simulink model "LKAS_AutoSave_DF_20220125_0841"  (R2018b)
settings: Solver=FixedStepDiscrete  StartTime=0.0  StopTime=10.0  FixedStep=0.01  RelTol=1e-3
InitFcn:
  | tmpVer = ver('MATLAB');
  | tmpVer = str2num(tmpVer.Version);
  | % -------------------------------------------------------------------
  | %  MATLAB file generated by Simulink.saveVars on 21-Nov-2019 10:06:14
  | %  MATLAB version: 7.13.0.564 (R2011b)
  | % -------------------------------------------------------------------
  | 
  | 
  | SInt16 = Simulink.AliasType;
  | SInt16.Description = 'Num';
  | if (tmpVer > 7.11)
  | 	SInt16.DataScope = 'Auto';
  | end
  | SInt16.HeaderFile = 'Rte_Type.h';
  | SInt16.BaseType = 'int16';
  | 
  | SInt32 = Simulink.AliasType;
  | SInt32.Description = 'Num';
  | if (tmpVer > 7.11)
  | 	SInt32.DataScope = 'Auto';
  | end
  | SInt32.HeaderFile = 'Rte_Type.h';
  | SInt32.BaseType = 'int32';
  | 
  | SInt8 = Simulink.AliasType;
  | SInt8.Description = 'Num';
  | if (tmpVer > 7.11)
  | 	SInt8.DataScope = 'Auto';
  | end
  | SInt8.HeaderFile = 'Rte_Type.h';
  | SInt8.BaseType = 'int8';
  | 
  | T_A_m2_1024_1_u32 = Simulink.NumericType;
  | T_A_m2_1024_1_u32.Description = 'm2 (square meters  (m2))';
  | if (tmpVer > 7.11)
  | 	T_A_m2_1024_1_u32.DataScope = 'Auto';
  | end
  | T_A_m2_1024_1_u32.HeaderFile = 'Rte_Type.h';
  | T_A_m2_1024_1_u32.DataTypeMode = 'Fixed-point: slope and bias scaling';
  | T_A_m2_1024_1_u32.SignednessBool = false;
  | T_A_m2_1024_1_u32.WordLength = 32;
  | T_A_m2_1024_1_u32.FixedExponent = -10;
  | T_A_m2_1024_1_u32.SlopeAdjustmentFactor = 1;
  | T_A_m2_1024_1_u32.Bias = 0;
  | T_A_m2_1024_1_u32.DataTypeOverride = 'Inherit';
  | T_A_m2_1024_1_u32.IsAlias = true;
  | 
  | T_A_m2_65536_1_u16 = Simulink.NumericType;
  | T_A_m2_65536_1_u16.Description = 'm2 (square meters  (m2))';
  | if (tmpVer > 7.11)
  | 	T_A_m2_65536_1_u16.DataScope = 'Auto';
  | end
  | T_A_m2_65536_1_u16.HeaderFile = 'Rte_Type.h';
  | T_A_m2_65536_1_u16.DataTypeMode = 'Fixed-point: slope and bias scaling';
  | T_A_m2_65536_1_u16.SignednessBool = false;
  | T_A_m2_65536_1_u16.WordLength = 16;
  | T_A_m2_65536_1_u16.FixedExponent = -16;
  | T_A_m2_65536_1_u16.SlopeAdjustmentFactor = 1;
  | T_A_m2_65536_1_u16.Bias = 0;
  | T_A_m2_65536_1_u16.DataTypeOverride = 'Inherit';
  | ... (+4647 lines)
StopFcn:
  | clear  T_A_m2_1024_1_u32 T_A_m2_65536_1_u16 T_A_m2_Float32 T_A_mm2_10_1_u16 T_A_mm2_4_1_s16 T_A_mm2_Float32 T_Cnt_Num_10_1_u32 T_Cnt_Num_1_1_s16 T_Cnt_Num_1_1_s32 T_Cnt_Num_1_1_s8 T_Cnt_Num_1_1_u16 T_Cnt_Num_1_1_u32 T_Cnt_Num_1_1_u8 T_E_J_1_1_s32 T_E_J_Float32 T_E_kJ_128_1_s32 T_E_kJ_Float32 T_E_kwh_10_1_u16 T_E_kwh_Float32 T_Epl_kwhpkm_100_1_u16 T_Epl_kwhpkm_Float32 T_F_N_1_1_s16 T_F_N_Float32 T_I_A_1000_1_u16 T_I_A_1048576_1_s32 T_I_A_2048_1_s16 T_I_A_32_1_s16 T_I_A_Float32 T_I_mA_1_1_s16 T_I_mA_32768_128_s16 T_I_mA_Float32 T_J_kgpm2_128_1_u16 T_J_kgpm2_Float32 T_K_NA_1000_1_s16 T_K_NA_100_1_s16 T_K_NA_100_1_u16 T_K_NA_1024_1_s16 T_K_NA_1024_1_u16 T_K_NA_128_1_s16 T_K_NA_128_1_u16 T_K_NA_128_1_u8 T_K_NA_16777216_1_u32 T_K_NA_16_1_s16 T_K_NA_16_1_u16 T_K_NA_16_1_u8 T_K_NA_1_16_u16 T_K_NA_1_1_s16 T_K_NA_1_1_u16 T_K_NA_1_1_u8 T_K_NA_32768_1_s16 T_K_NA_32768_1_u16 T_K_NA_32_1_s8 T_K_NA_4096_1_u16 T_K_NA_4194304_1_s32 T_K_NA_4194304_1_u16 T_K_NA_65536_1_s32 T_K_NA_65536_1_u16 T_K_NA_8192_1_s16 T_K_NA_8_1_s16 T_K_NA_Float32 T_M_Nm_16_1_s16 T_M_Nm_1_1_s16 T_M_Nm_32768_1_s16 T_M_Nm_32_1_s16 T_M_Nm_4_1_s16 T_M_Nm_512_1_s16 T_M_Nm_Float32 T_P_W_1_4_s16 T_P_W_1_8_s16 T_P_W_Float32 T_P_kW_128_1_s16 T_P_kW_1_8_s16 T_P_kW_8_1_s32 T_P_kW_Float32 T_Pct_pct_1024_1_s32 T_Pct_pct_1024_1_u32 T_Pct_pct_10_1_s16 T_Pct_pct_10_1_u32 T_Pct_pct_128_100_s8 T_Pct_pct_1_1_s16 T_Pct_pct_1_4_u8 T_Pct_pct_255_100_u16 T_Pct_pct_255_100_u8 T_Pct_pct_256_1_s16 T_Pct_pct_256_1_u16 T_Pct_pct_65535_100_u16 T_Pct_pct_Float32 T_R_ohm_1024_1_s16 T_R_ohm_32_1_s16 T_R_ohm_Float32 T_TK_K_16_1_s16 T_TK_K_Float32 T_T_degC_10_400_1_u16 T_T_degC_16_1_s16 T_T_degC_1_40_1_u8 T_T_degC_2_80_1_u8 T_T_degC_Float32 T_U_V_1000_1_u16 T_U_V_10_1_u8 T_U_V_200_1_u8 T_U_V_32_1_s16 T_U_V_4096_1_s16 T_U_V_512_1_s16 T_U_V_65535_8_u16 T_U_V_8192_1_u16 T_U_V_Float32 T_U_mV_1_1_s16 T_U_mV_256_20_u16 T_U_mV_Float32 T_V_l_256_1_s16 T_V_l_4096_1_s16 T_V_l_64_1_s16 T_V_l_65535_100_u16 T_V_l_Float32 T_V_ml_128_1_s16 T_V_ml_1_1_s16 T_V_ml_32768_1_s16 T_V_ml_Float32 T_V_ul_32_1_u16 T_V_ul_Float32 T_Vpl_clpkm_512_1_u16 T_Vpl_clpkm_Float32 T_a_kphps_16_1_s16 T_a_kphps_Float32 T_a_mps2_128_1_s16 T_a_mps2_Float32 T_c_MJpkg_256_1_s16 T_c_MJpkg_Float32 T_c_kJpgpK_1024_1_s16 T_c_kJpgpK_Float32 T_c_kJpkgpK_128_1_u16 T_c_kJpkgpK_Float32 T_chrg_Ah_1_1_s16 T_chrg_Ah_1_1_u16 T_chrg_Ah_1_1_u8 T_chrg_Ah_256_1_u16 T_chrg_Ah_4194304_1_s32 T_chrg_Ah_512_1_u16 T_chrg_Ah_8_1_u16 T_chrg_Ah_Float32 T_cmp_NA_100_1_s16 T_cmp_NA_128_1_s16 T_cmp_NA_16_1_s16 T_cmp_NA_32768_1_u16 T_cmp_NA_Float32 T_d2n_rpmps2_4_1_s16 T_d2n_rpmps2_Float32 T_dPct_pctps_16_1_s16 T_dPct_pctps_256_1_s16 T_dPct_pctps_Float32 T_dT_degCps_128_1_s16 T_dT_degCps_Float32 T_dV_lph_1_1_s16 T_dV_lph_Float32 T_dV_lpm_128_1_s16 T_dV_lpm_32_1_s16 T_dV_lpm_Float32 T_dV_lps_1024_1_u16 T_dV_lps_4_1_u16 T_dV_lps_Float32 T_dV_mlps_1024_1_s16 T_dV_mlps_Float32 T_d_BitField16 T_dm_gps_128_1_s16 T_dm_gps_128_1_u16 T_dm_gps_256_1_u16 T_dm_gps_Float32 T_dm_mgps_1_1_s16 T_dm_mgps_Float32 T_dn_rpmps_1_1_s16 T_dn_rpmps_2_1_s16 T_dn_rpmps_Float32 T_dp_Paps_1_1_s16 T_dp_Paps_Float32 T_dp_kPaps_1_1_s16 T_dp_kPaps_8_1_s16 T_dp_kPaps_Float32 T_dphi_degps_128_1_s16 T_dphi_degps_8_1_s16 T_dphi_degps_Float32 T_dr_ps_256_1_s16 T_dr_ps_Float32 T_drho_mgplps_1_2_s16 T_drho_mgplps_Float32 T_e_NA_1_1_u8 T_f_Hz_1_1_u16 T_f_Hz_1_1_u32 T_f_Hz_64_1_u16 T_f_Hz_8_1_s16 T_f_Hz_Float32 T_g_BitField32 T_l_km_16_1_s16 T_l_km_1_1_u16 T_l_km_1_1_u32 T_l_km_Float32 T_l_m_1024_1_s16 T_l_m_16_1_s16 T_l_m_1_1_u32 T_l_m_Float32 T_l_mm_16_1_s16 T_l_mm_1_1_u16 T_l_mm_4096_1_s16 T_l_mm_4_1_u8 T_l_mm_64_1_s16 T_l_mm_Float32 T_m_g_1_1_s16 T_m_g_2048_1_s16 T_m_g_32_1_u16 T_m_g_Float32 T_m_kg_1024_1_s16 T_m_kg_1_1_s16 T_m_kg_1_1_u32 T_m_kg_Float32 T_m_mg_128_1_s16 T_m_mg_32_1_s16 T_m_mg_Float32 T_n_rpm_1_1_s16 T_n_rpm_1_25_u8 T_n_rpm_256_50_u16 T_n_rpm_2_25_u8 T_n_rpm_4_1_u16 T_n_rpm_Float32 T_p_MPa_64_1_s16 T_p_MPa_Float32 T_p_Pa_1_1_s16 T_p_Pa_Float32 T_p_kPa_1_10_u16 T_p_kPa_1_1_s16 T_p_kPa_1_1_u8 T_p_kPa_256_1_u16 T_p_kPa_32_1_u16 T_p_kPa_64_1_s16 T_p_kPa_Float32 T_phi_deg_100_1_s16 T_phi_deg_1024_1_s16 T_phi_deg_128_1_s16 T_phi_deg_1_1_u8 T_phi_deg_256_1_s16 T_phi_deg_2_1_s8 T_phi_deg_32_1_s16 T_phi_deg_512_6_s32 T_phi_deg_Float32 T_phi_rad_2048_1_s16 T_phi_rad_Float32 T_r_NA_1024_1_s16 T_r_NA_1024_1_u16 T_r_NA_16384_1_s16 T_r_NA_16_1_s16 T_r_NA_256_1_s8 T_r_NA_256_1_u16 T_r_NA_32768_1_u16 T_r_NA_32_1_u16 T_r_NA_4096_1_s16 T_r_NA_65535_2_u16 T_r_NA_8192_1_u16 T_r_NA_Float32 T_rho_gpl_8192_1_s16 T_rho_gpl_Float32 T_rho_kgpm3_16_1_s16 T_rho_kgpm3_Float32 T_rho_mgpl_1_1_s16 T_rho_mgpl_64_1_s16 T_rho_mgpl_Float32 T_t_hour_1_1_s16 T_t_hour_Float32 T_t_m_1_1_u16 T_t_m_Float32 T_t_ms_1_1_s16 T_t_ms_1_1_u16 T_t_ms_1_1_u32 T_t_ms_4096_1_s16 T_t_ms_64_1_s16 T_t_ms_Float32 T_t_s_1000_1_s16 T_t_s_100_1_s16 T_t_s_10_1_s16 T_t_s_10_1_u16 T_t_s_1_1_s16 T_t_s_1_1_u16 T_t_s_1_1_u32 T_t_s_Float32 T_t_us_10_1_u32 T_t_us_1_1_s16 T_t_us_1_1_u32 T_t_us_1_4_u16 T_t_us_Float32 T_v_kph_1_1_u8 T_v_kph_64_1_s16 T_v_kph_64_1_u16 T_v_kph_Float32 T_v_mps_256_1_s16 T_v_mps_Float32 T_w_radps_32_1_s16 T_w_radps_Float32 T_y_BitField8 T_y_BitFieldDiagProgress T_y_BitFieldDiagStatus T_y_NA_1_1_u8 SInt16 SInt32 SInt8 T_BOOLEAN UInt16 UInt32 UInt8 s16 s32 s8 u16 u32 u8
model workspace (MAT data in the model file):
  MCOS : class17 (value not decoded)
  MCOS : class17 (value not decoded)
  MCOS : class17 (value not decoded)
  MCOS : class17 (value not decoded)
  MCOS : class17 (value not decoded)
  MCOS : class17 (value not decoded)
  MCOS : class17 (value not decoded)
  MCOS : class17 (value not decoded)
  MCOS : class17 (value not decoded)
  MCOS : class17 (value not decoded)
  MCOS : class17 (value not decoded)
  MCOS : class17 (value not decoded)
  MCOS : class17 (value not decoded)
  MCOS : class17 (value not decoded)
  MCOS : class17 (value not decoded)
  MCOS : class17 (value not decoded)
  MCOS : class17 (value not decoded)
  MCOS : class17 (value not decoded)
  MCOS : class17 (value not decoded)
  MCOS : class17 (value not decoded)
  MCOS : class17 (value not decoded)
  MCOS : class17 (value not decoded)
  MCOS : class17 (value not decoded)
  MCOS : class17 (value not decoded)
  MCOS : class17 (value not decoded)
  MCOS : class17 (value not decoded)
  MCOS : class17 (value not decoded)
  MCOS : class17 (value not decoded)
  MCOS : class17 (value not decoded)
  MCOS : class17 (value not decoded)
  MCOS : class17 (value not decoded)
  MCOS : class17 (value not decoded)
  MCOS : class17 (value not decoded)
  MCOS : class17 (value not decoded)
  MCOS : class17 (value not decoded)
  MCOS : class17 (value not decoded)
  MCOS : class17 (value not decoded)
  MCOS : class17 (value not decoded)
  MCOS : class17 (value not decoded)
  MCOS : class17 (value not decoded)
  MCOS : class17 (value not decoded)
  MCOS : class17 (value not decoded)
  MCOS : class17 (value not decoded)
  MCOS : class17 (value not decoded)
  MCOS : class17 (value not decoded)
  MCOS : class17 (value not decoded)
  MCOS : class17 (value not decoded)
  MCOS : class17 (value not decoded)
  MCOS : class17 (value not decoded)
  MCOS : class17 (value not decoded)
  MCOS : class17 (value not decoded)
  MCOS : class17 (value not decoded)
  MCOS : class17 (value not decoded)
  MCOS : class17 (value not decoded)
  MCOS : class17 (value not decoded)
  MCOS : class17 (value not decoded)
  MCOS : class17 (value not decoded)
  MCOS : class17 (value not decoded)
  MCOS : class17 (value not decoded)
  MCOS : class17 (value not decoded)
  MCOS : class17 (value not decoded)
  MCOS : class17 (value not decoded)
  MCOS : class17 (value not decoded)
  MCOS : class17 (value not decoded)
  MCOS : class17 (value not decoded)
  MCOS : class17 (value not decoded)
  MCOS : class17 (value not decoded)
  MCOS : class17 (value not decoded)
  MCOS : class17 (value not decoded)
  MCOS : class17 (value not decoded)
  MCOS : class17 (value not decoded)
  MCOS : class17 (value not decoded)
  MCOS : class17 (value not decoded)
  MCOS : class17 (value not decoded)
  MCOS : class17 (value not decoded)
  MCOS : class17 (value not decoded)
  MCOS : class17 (value not decoded)
  MCOS : class17 (value not decoded)
  MCOS : class17 (value not decoded)
  MCOS : class17 (value not decoded)
  MCOS : class17 (value not decoded)
  MCOS : class17 (value not decoded)
  MCOS : class17 (value not decoded)
  MCOS : class17 (value not decoded)
  MCOS : class17 (value not decoded)
  MCOS : class17 (value not decoded)
  MCOS : class17 (value not decoded)
  MCOS : class17 (value not decoded)
  MCOS : class17 (value not decoded)
  MCOS : class17 (value not decoded)
  MCOS : class17 (value not decoded)
  MCOS : class17 (value not decoded)
  MCOS : class17 (value not decoded)
  MCOS : class17 (value not decoded)
  MCOS : class17 (value not decoded)
  MCOS : class17 (value not decoded)
  MCOS : class17 (value not decoded)
  MCOS : class17 (value not decoded)
  MCOS : class17 (value not decoded)
  MCOS : class17 (value not decoded)
  MCOS : class17 (value not decoded)
  MCOS : class17 (value not decoded)
undefined symbols (not defined in the file): LKA_CarWidth, LKA_SampleTime, LKA_StrRatio_C, LKA_Veh2CamL_C, LKA_Veh2CamW_C, LKA_WhlBaseL_C, LL_CompHdAg_C, LL_CompSWA_C, LL_CrvtPrvwT_C, LL_DesDvt_C, LL_DvtComp_C, LL_DvtPrvwT_C, LL_DvtSpdDet_vDvtSpdMin_C, LL_HandsOff_ExitTime, LL_HandsOff_TextTime, LL_HandsOff_WarnTime, LL_HdAgExT_C, LL_HdAgPrvwT_C, LL_LAccMax_C, LL_LAccRMax_C, LL_LDW_EarliestWarnLine_C, LL_LDW_LatestWarnLine_C, LL_LDWS_SUPPRESS_HEADING, LL_LFClb_TFC_FfCtlRatio_C, LL_LFClb_TFC_KdBalance_C, LL_LFClb_TFC_KdMaxSWA_C, LL_LFClb_TFC_KdV1_C, LL_LFClb_TFC_KdV2_C, LL_LFClb_TFC_KdVehSpdLwr_C, LL_LFClb_TFC_KdVehSpdUpr_C, LL_LFClb_TFC_Ki_C, LL_LFClb_TFC_KiMaxSWA_C, LL_LFClb_TFC_Kp_C, LL_LFClb_TFC_KpKlat_C, LL_LFClb_TFC_KpV1_C, LL_LFClb_TFC_KpV2_C, LL_LFClb_TFC_KpVehSpdLwr_C, LL_LFClb_TFC_KpVehSpdUpr_C, LL_LFClb_TFC_PrvwT_C, LL_LKA_EarliestWarnLine_C, LL_LKA_LatestWarnLine_C, LL_LKAExPrcs_ExitC0Dvt, LL_LKAExPrcs_ExitC0Swt, LL_LKAExPrcs_tiExitTime1, LL_LKAExPrcs_tiExitTime2, LL_LKAExPrcs_tiExitTime3, LL_LKAS_OUT_OF_CONTROL_LAT_VEL, LL_LKAS_OUT_OF_CONTROL_TTLC, LL_LKASWASyn_M0, LL_LKASWASyn_M1, LL_LKASWASyn_M2, LL_LKASWASyn_M3K, LL_LKASWASyn_SWAaddMax, LL_LKASWASyn_T2, LL_LKASWASyn_tiTrqSwaRtTime, LL_LKASWASyn_tiTrqSwaTime, LL_LKASWASyn_TrqMax, LL_LKASWASyn_TrqSwaAddSwt, LL_LKASWASyn_TrqSwaRateDiff, LL_LSpdCompT_C ... (+43)
libraries: simulink x136, canmsglib x8, dspstat3 x3, simulink_extras x1
(part 12 of 20)

== system LKAS_AutoSave_DF_20220125_0841/LKAS/LL/LLOn/LKA/LKA Motion Planning (LKAMP) /LKA Motion Planning Calculation (LKAMPCal)/Time Division (TDiv)3 ==
  TDiv_bsTDivInfoOut1 : Inport
  Add : Sum  OutDataTypeStr=uint16
  Constant : Constant  OutDataTypeStr=uint16  SampleTime=-1
  Constant19 : Constant  OutDataTypeStr=uint16  SampleTime=-1
  If : If  NumInputs=2  IfExpression=u1==u2
  Memory : Memory  InheritSampleTime=on
  Merge1 : Merge
  Saturation1 : Saturate  UpperLimit=100  LowerLimit=0  OutDataTypeStr=uint16
      settings: AttributesFormatString="Min = %<LowerLimit>  Max = %<UpperLimit>"
  if action 3 : Subsystem  TreatAsAtomicUnit=on
  if action 4 : Subsystem  TreatAsAtomicUnit=on
  Out2 : Outport
  wires:
  Merge1/1 -> Out2/1
  TDiv_bsTDivInfoOut1/1 -> if action 3/1(In1)
  if action 4/1(Out1) -> Merge1/1
  if action 3/1(Out1) -> Merge1/2
  If/2 -> if action 3/Action
  Saturation1/1 -> If/1
  Add/1 -> Saturation1/1, Memory/1
  Constant19/1 -> If/2
  Constant/1 -> Add/1
  Memory/1 -> Add/2
  If/1 -> if action 4/Action

== system LKAS_AutoSave_DF_20220125_0841/LKAS/LL/LLOn/LKA/LKA Motion Planning (LKAMP) /LKA Motion Planning Calculation (LKAMPCal)/Time Division (TDiv)4 ==
  TDiv_bsTDivInfoOut1 : Inport
  Add : Sum  OutDataTypeStr=uint16
  Constant : Constant  OutDataTypeStr=uint16  SampleTime=-1
  Constant19 : Constant  OutDataTypeStr=uint16  SampleTime=-1
  If : If  NumInputs=2  IfExpression=u1==u2
  Memory : Memory  InheritSampleTime=on
  Merge1 : Merge
  Saturation1 : Saturate  UpperLimit=100  LowerLimit=0  OutDataTypeStr=uint16
      settings: AttributesFormatString="Min = %<LowerLimit>  Max = %<UpperLimit>"
  if action 3 : Subsystem  TreatAsAtomicUnit=on
  if action 4 : Subsystem  TreatAsAtomicUnit=on
  Out2 : Outport
  wires:
  If/1 -> if action 4/Action
  Memory/1 -> Add/2
  Constant/1 -> Add/1
  Constant19/1 -> If/2
  Add/1 -> Memory/1, Saturation1/1
  Saturation1/1 -> If/1
  If/2 -> if action 3/Action
  if action 3/1(Out1) -> Merge1/2
  if action 4/1(Out1) -> Merge1/1
  TDiv_bsTDivInfoOut1/1 -> if action 3/1(In1)
  Merge1/1 -> Out2/1

== system LKAS_AutoSave_DF_20220125_0841/LKAS/LL/LLOn/LKA/LKA Motion Planning (LKAMP) /Motion Planning Input Processing (MPInP)/Lane Information Selection (LaneInfoSel) ==
  LaneInfoSel_stLKAActvFlg : Inport
  LaneInfoSel_facmLftLane : Inport  Port=2
  LaneInfoSel_facmRgtLane : Inport  Port=3
  If : If  IfExpression=u1==1  ElseIfExpressions=u1==2
  If Action Subsystem1 : Subsystem  TreatAsAtomicUnit=on
  If Action Subsystem2 : Subsystem  TreatAsAtomicUnit=on
  If Action Subsystem3 : Subsystem  TreatAsAtomicUnit=on
  Merge : Merge  Inputs=3
  LaneInfoSel_facmActvLane : Outport
  wires:
  LaneInfoSel_facmRgtLane/1 -> If Action Subsystem1/1(In1)
  LaneInfoSel_facmLftLane/1 -> If Action Subsystem2/1(In1)
  LaneInfoSel_stLKAActvFlg/1 -> If/1
  If/1 -> If Action Subsystem2/Action
  If Action Subsystem2/1(Out1) -> Merge/1
  Merge/1 -> LaneInfoSel_facmActvLane/1
  If/2 -> If Action Subsystem1/Action
  If Action Subsystem1/1(Out1) -> Merge/2
  If Action Subsystem3/1(Out1) -> Merge/3
  If/3 -> If Action Subsystem3/Action

== system LKAS_AutoSave_DF_20220125_0841/LKAS/LL/LLOn/LKA/LKA Motion Planning (LKAMP) /Motion Planning Input Processing (MPInP)/Lane Information Selection (LaneInfoSel)1 ==
  LaneInfoSel_stLKAActvFlg : Inport
  LaneInfoSel_facmLftLane : Inport  Port=2
  LaneInfoSel_facmRgtLane : Inport  Port=3
  If : If  IfExpression=u1==1  ElseIfExpressions=u1==2
  If Action Subsystem1 : Subsystem  TreatAsAtomicUnit=on
  If Action Subsystem2 : Subsystem  TreatAsAtomicUnit=on
  If Action Subsystem3 : Subsystem  TreatAsAtomicUnit=on
  Merge : Merge  Inputs=3
  LaneInfoSel_facmActvLane : Outport
  wires:
  LaneInfoSel_facmRgtLane/1 -> If Action Subsystem1/1(In1)
  LaneInfoSel_facmLftLane/1 -> If Action Subsystem2/1(In1)
  LaneInfoSel_stLKAActvFlg/1 -> If/1
  If/1 -> If Action Subsystem2/Action
  If Action Subsystem2/1(Out1) -> Merge/1
  Merge/1 -> LaneInfoSel_facmActvLane/1
  If/2 -> If Action Subsystem1/Action
  If Action Subsystem1/1(Out1) -> Merge/2
  If Action Subsystem3/1(Out1) -> Merge/3
  If/3 -> If Action Subsystem3/Action

== system LKAS_AutoSave_DF_20220125_0841/LKAS/LL/LLOn/LKA/LKA Motion Planning (LKAMP) /Motion Planning Input Processing (MPInP)/Lane Information Selection (LaneInfoSel)2 ==
  LaneInfoSel_stLKAActvFlg : Inport
  LaneInfoSel_facmLftLane : Inport  Port=2
  LaneInfoSel_facmRgtLane : Inport  Port=3
  If : If  IfExpression=u1==1  ElseIfExpressions=u1==2
  If Action Subsystem1 : Subsystem  TreatAsAtomicUnit=on
  If Action Subsystem2 : Subsystem  TreatAsAtomicUnit=on
  If Action Subsystem3 : Subsystem  TreatAsAtomicUnit=on
  Merge : Merge  Inputs=3
  LaneInfoSel_facmActvLane : Outport
  wires:
  LaneInfoSel_facmRgtLane/1 -> If Action Subsystem1/1(In1)
  LaneInfoSel_facmLftLane/1 -> If Action Subsystem2/1(In1)
  LaneInfoSel_stLKAActvFlg/1 -> If/1
  If/1 -> If Action Subsystem2/Action
  If Action Subsystem2/1(Out1) -> Merge/1
  Merge/1 -> LaneInfoSel_facmActvLane/1
  If/2 -> If Action Subsystem1/Action
  If Action Subsystem1/1(Out1) -> Merge/2
  If Action Subsystem3/1(Out1) -> Merge/3
  If/3 -> If Action Subsystem3/Action

== system LKAS_AutoSave_DF_20220125_0841/LKAS/LL/LLOn/LKA/LKA Motion Planning (LKAMP) /Motion Planning Input Processing (MPInP)/Signal Latching ==
  In : Inport
  Add : Sum  OutDataTypeStr=uint16
  Constant : Constant  OutDataTypeStr=uint16  SampleTime=-1
  Constant2 : Constant  Value=LatchTime  OutDataTypeStr=uint16  SampleTime=-1
  If : If  NumInputs=2  IfExpression=u1==u2  ShowElse=off
  Memory : Memory  InheritSampleTime=on
  Saturation1 : Saturate  UpperLimit=10000  LowerLimit=0  OutDataTypeStr=uint16
  "if action " : Subsystem  TreatAsAtomicUnit=on
  Out : Outport
  wires:
  Constant2/1 -> If/2
  In/1 -> "if action "/1(In)
  "if action "/1(Out) -> Out/1
  If/1 -> "if action "/Action
  Constant/1 -> Add/1
  Add/1 -> Memory/1, Saturation1/1
  Memory/1 -> Add/2
  Saturation1/1 -> If/1

== system LKAS_AutoSave_DF_20220125_0841/LKAS/LL/LLOn/LKA/LKA Motion Planning (LKAMP) /Motion Planning Input Processing (MPInP)/Signal Latching2 ==
  In : Inport
  Add : Sum  OutDataTypeStr=uint16
  Constant : Constant  OutDataTypeStr=uint16  SampleTime=-1
  Constant2 : Constant  Value=LatchTime  OutDataTypeStr=uint16  SampleTime=-1
  If : If  NumInputs=2  IfExpression=u1==u2  ShowElse=off
  Memory : Memory  InheritSampleTime=on
  Saturation1 : Saturate  UpperLimit=10000  LowerLimit=0  OutDataTypeStr=uint16
  "if action " : Subsystem  TreatAsAtomicUnit=on
  Out : Outport
  wires:
  Constant2/1 -> If/2
  In/1 -> "if action "/1(In)
  "if action "/1(Out) -> Out/1
  If/1 -> "if action "/Action
  Constant/1 -> Add/1
  Add/1 -> Saturation1/1
  Memory/1 -> Add/2
  Saturation1/1 -> Memory/1, If/1

== system LKAS_AutoSave_DF_20220125_0841/LKAS/LL/LLOn/LKA/LKA Motion Planning (LKAMP) /Motion Planning Input Processing (MPInP)/Signal Latching3 ==
  In : Inport
  Add : Sum  OutDataTypeStr=uint16
  Constant : Constant  OutDataTypeStr=uint16  SampleTime=-1
  Constant2 : Constant  Value=LatchTime  OutDataTypeStr=uint16  SampleTime=-1
  If : If  NumInputs=2  IfExpression=u1==u2  ShowElse=off
  Memory : Memory  InheritSampleTime=on
  Saturation1 : Saturate  UpperLimit=10000  LowerLimit=0  OutDataTypeStr=uint16
  "if action " : Subsystem  TreatAsAtomicUnit=on
  Out : Outport
  wires:
  Saturation1/1 -> If/1, Memory/1
  Memory/1 -> Add/2
  Add/1 -> Saturation1/1
  Constant/1 -> Add/1
  If/1 -> "if action "/Action
  "if action "/1(Out) -> Out/1
  In/1 -> "if action "/1(In)
  Constant2/1 -> If/2

== system LKAS_AutoSave_DF_20220125_0841/LKAS/LL/LLOn/LKA/LKA Motion Planning (LKAMP) /Motion Planning Input Processing (MPInP)/Signal Latching4 ==
  In : Inport
  Add : Sum  OutDataTypeStr=uint16
  Constant : Constant  OutDataTypeStr=uint16  SampleTime=-1
  Constant2 : Constant  Value=LatchTime  OutDataTypeStr=uint16  SampleTime=-1
  If : If  NumInputs=2  IfExpression=u1==u2  ShowElse=off
  Memory : Memory  InheritSampleTime=on
  Saturation1 : Saturate  UpperLimit=10000  LowerLimit=0  OutDataTypeStr=uint16
  "if action " : Subsystem  TreatAsAtomicUnit=on
  Out : Outport
  wires:
  Constant2/1 -> If/2
  In/1 -> "if action "/1(In)
  "if action "/1(Out) -> Out/1
  If/1 -> "if action "/Action
  Constant/1 -> Add/1
  Add/1 -> Saturation1/1
  Memory/1 -> Add/2
  Saturation1/1 -> Memory/1, If/1

== system LKAS_AutoSave_DF_20220125_0841/LKAS/LL/LLOn/LKA/LKA Motion Planning (LKAMP) /Motion Planning Input Processing (MPInP)/Signal Latching5 ==
  In : Inport
  Add : Sum  OutDataTypeStr=uint16
  Constant : Constant  OutDataTypeStr=uint16  SampleTime=-1
  Constant2 : Constant  Value=LatchTime  OutDataTypeStr=uint16  SampleTime=-1
  If : If  NumInputs=2  IfExpression=u1==u2  ShowElse=off
  Memory : Memory  InheritSampleTime=on
  Saturation1 : Saturate  UpperLimit=10000  LowerLimit=0  OutDataTypeStr=uint16
  "if action " : Subsystem  TreatAsAtomicUnit=on
  Out : Outport
  wires:
  Constant2/1 -> If/2
  In/1 -> "if action "/1(In)
  "if action "/1(Out) -> Out/1
  If/1 -> "if action "/Action
  Constant/1 -> Add/1
  Add/1 -> Saturation1/1
  Memory/1 -> Add/2
  Saturation1/1 -> Memory/1, If/1

== system LKAS_AutoSave_DF_20220125_0841/LKAS/LL/LLOn/LKA/LKA Motion Planning (LKAMP) /Motion Planning Input Processing (MPInP)/Signal Latching6 ==
  In : Inport
  Add : Sum  OutDataTypeStr=uint16
  Constant : Constant  OutDataTypeStr=uint16  SampleTime=-1
  Constant2 : Constant  Value=LatchTime  OutDataTypeStr=uint16  SampleTime=-1
  If : If  NumInputs=2  IfExpression=u1==u2  ShowElse=off
  Memory : Memory  InheritSampleTime=on
  Saturation1 : Saturate  UpperLimit=10000  LowerLimit=0  OutDataTypeStr=uint16
  "if action " : Subsystem  TreatAsAtomicUnit=on
  Out : Outport
  wires:
  Constant2/1 -> If/2
  In/1 -> "if action "/1(In)
  "if action "/1(Out) -> Out/1
  If/1 -> "if action "/Action
  Constant/1 -> Add/1
  Add/1 -> Saturation1/1
  Memory/1 -> Add/2
  Saturation1/1 -> Memory/1, If/1

== system LKAS_AutoSave_DF_20220125_0841/LKAS/LL/LLOn/LKA/LKA Motion Planning (LKAMP) /Motion Planning Input Processing (MPInP)/Signal Latching7 ==
  In : Inport
  Add : Sum  OutDataTypeStr=uint16
  Constant : Constant  OutDataTypeStr=uint16  SampleTime=-1
  Constant2 : Constant  Value=LatchTime  OutDataTypeStr=uint16  SampleTime=-1
  If : If  NumInputs=2  IfExpression=u1==u2  ShowElse=off
  Memory : Memory  InheritSampleTime=on
  Saturation1 : Saturate  UpperLimit=10000  LowerLimit=0  OutDataTypeStr=uint16
  "if action " : Subsystem  TreatAsAtomicUnit=on
  Out : Outport
  wires:
  Saturation1/1 -> If/1, Memory/1
  Memory/1 -> Add/2
  Add/1 -> Saturation1/1
  Constant/1 -> Add/1
  If/1 -> "if action "/Action
  "if action "/1(Out) -> Out/1
  In/1 -> "if action "/1(In)
  Constant2/1 -> If/2

== system LKAS_AutoSave_DF_20220125_0841/LKAS/LL/LLOn/LKA/LKA Motion Planning (LKAMP) /Motion Planning Input Processing (MPInP)/Subsystem ==
  In1 : Inport
  If : If  IfExpression=u1==1  ElseIfExpressions=u1==2
  If Action Subsystem1 : Subsystem  TreatAsAtomicUnit=on
  If Action Subsystem2 : Subsystem  TreatAsAtomicUnit=on
  If Action Subsystem3 : Subsystem  TreatAsAtomicUnit=on
  Merge : Merge  Inputs=3
  Out6 : Outport
  wires:
  If/3 -> If Action Subsystem3/Action
  If Action Subsystem3/1(Out1) -> Merge/3
  If Action Subsystem1/1(Out1) -> Merge/2
  If/2 -> If Action Subsystem1/Action
  Merge/1 -> Out6/1
  If Action Subsystem2/1(Out1) -> Merge/1
  If/1 -> If Action Subsystem2/Action
  In1/1 -> If/1

== system LKAS_AutoSave_DF_20220125_0841/LKAS/LL/LLOn/LKA/LKA Motion Planning (LKAMP) /Switching Condition (SwtCon)/Ending Heading Angle Determination (EndHdAgDet) ==
  EndHdAgDet_stLKAActvFlg : Inport
  EndHdAgDet_vVehSpd : Inport  Port=2
  EndHdAgDet_crPrvwCrvt : Inport  Port=3
  EndHdAgDet_lLaneWidth_C : Inport  Port=4
  EndHdAgDet_lCarWidth_C : Inport  Port=5
  EndHdAgDet_tiHdAgExTime_C : Inport  Port=6
  EndHdAgDet_tiLSpdCompT_C : Inport  Port=7
  Add : Sum  Inputs=+-  OutDataTypeStr=single
  Add1 : Sum  OutDataTypeStr=single
  Divide : Product  Inputs=/*  OutDataTypeStr=single
  Divide1 : Product  Inputs=*/  OutDataTypeStr=single
  Lateral Speed Compensation (LSpdComp) : Subsystem
  kph To mps : Gain  Gain=1/3.6  OutDataTypeStr=single
  EndHdAgDet_phiHdAgMax : Outport
  wires:
  EndHdAgDet_tiLSpdCompT_C/1 -> Lateral Speed Compensation (LSpdComp)/4(LSpdComp_tiLSpdCompT_C)
  EndHdAgDet_crPrvwCrvt/1 -> Lateral Speed Compensation (LSpdComp)/3(LSpdComp_crPrvwCrvt)
  Add1/1 -> EndHdAgDet_phiHdAgMax/1
  Divide1/1 -> Add1/1
  Lateral Speed Compensation (LSpdComp)/1(LSpdComp_phiLSpdComp) -> Add1/2
  Add/1 -> Divide/2
  EndHdAgDet_stLKAActvFlg/1 -> Lateral Speed Compensation (LSpdComp)/2(LSpdComp_stLKAFlg)
  EndHdAgDet_vVehSpd/1 -> kph To mps/1
  EndHdAgDet_tiHdAgExTime_C/1 -> Divide/1
  kph To mps/1 -> Divide1/2, Lateral Speed Compensation (LSpdComp)/1(LSpdComp_vVehSpd)
  EndHdAgDet_lCarWidth_C/1 -> Add/2
  EndHdAgDet_lLaneWidth_C/1 -> Add/1
  Divide/1 -> Divide1/1

== system LKAS_AutoSave_DF_20220125_0841/LKAS/LL/LLOn/LKA/LKA Motion Planning (LKAMP) /Switching Condition (SwtCon)/If Action Subsystem ==
  In1 : Inport
  Action Port : ActionPort  InitializeStates=reset
      settings: AttributesFormatString=states = %<InitializeStates>
  Gain2 : Gain  Gain=-1  OutDataTypeStr=Inherit: Same as input
  Out1 : Outport
      settings: AttributesFormatString=%<OutputWhenDisabled> = %<InitialOutput>
  wires:
  In1/1 -> Gain2/1
  Gain2/1 -> Out1/1  "HdAgMax"

== system LKAS_AutoSave_DF_20220125_0841/LKAS/LL/LLOn/LKA/LKA Motion Planning (LKAMP) /Switching Condition (SwtCon)/If Action Subsystem1 ==
  In1 : Inport
  Action Port : ActionPort  InitializeStates=reset
      settings: AttributesFormatString=states = %<InitializeStates>
  Cast To Single1 : DataTypeConversion  LockScale=on
  Out1 : Outport
      settings: AttributesFormatString=%<OutputWhenDisabled> = %<InitialOutput>
  wires:
  In1/1 -> Cast To Single1/1
  Cast To Single1/1 -> Out1/1  "HdAgMax"

== system LKAS_AutoSave_DF_20220125_0841/LKAS/LL/LLOn/LKA/LKA Motion Planning (LKAMP) /Switching Condition (SwtCon)/If Action Subsystem2 ==
  Action Port : ActionPort  InitializeStates=reset
      settings: AttributesFormatString=states = %<InitializeStates>
  Constant2 : Constant  Value=0  OutDataTypeStr=single  SampleTime=-1
  Out1 : Outport
      settings: AttributesFormatString=%<OutputWhenDisabled> = %<InitialOutput>
  wires:
  Constant2/1 -> Out1/1  "HdAgMax"

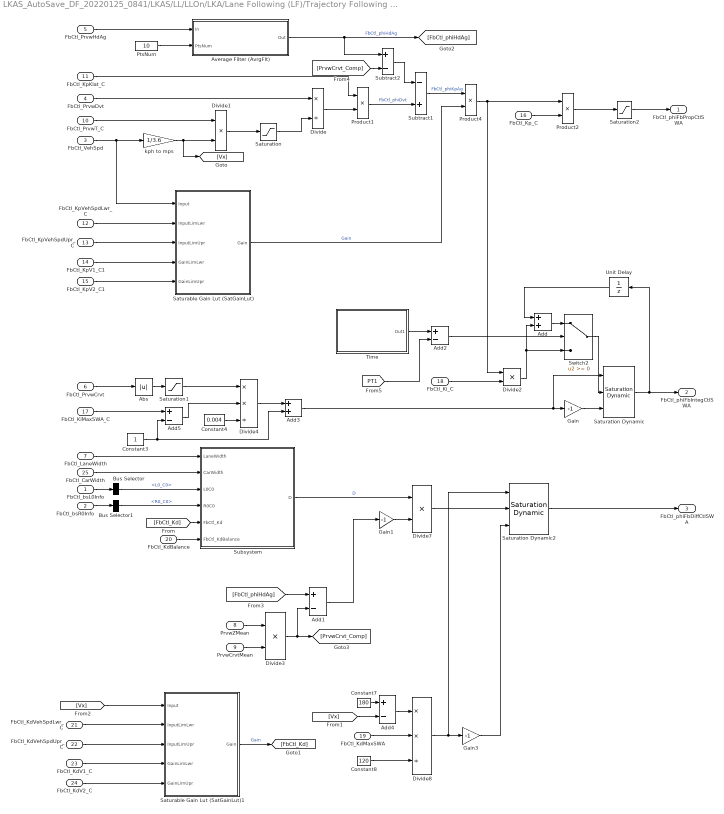
== system LKAS_AutoSave_DF_20220125_0841/LKAS/LL/LLOn/LKA/Lane Following (LF)/Trajectory Following Control (TFC)/Feedback Control (FbCtl) ==
  FbCtl_bsL0Info : Inport
  FbCtl_bsR0Info : Inport  Port=2
  FbCtl_VehSpd : Inport  Port=3
  FbCtl_PrvwDvt : Inport  Port=4
  FbCtl_PrvwHdAg : Inport  Port=5
  FbCtl_PrvwCrvt : Inport  Port=6
  FbCtl_LaneWidth : Inport  Port=7
  PrvwZMean : Inport  Port=8
  PrvwCrvtMean : Inport  Port=9
  FbCtl_PrvwT_C : Inport  Port=10
  FbCtl_KpKlat_C : Inport  Port=11
  FbCtl_KpVehSpdLwr_C : Inport  Port=12
  FbCtl_KpVehSpdUpr_C : Inport  Port=13
  FbCtl_KpV1_C1 : Inport  Port=14
  FbCtl_KpV2_C1 : Inport  Port=15
  FbCtl_Kp_C : Inport  Port=16
  FbCtl_KiMaxSWA_C : Inport  Port=17
  FbCtl_Ki_C : Inport  Port=18
  FbCtl_KdMaxSWA : Inport  Port=19
  FbCtl_KdBalance : Inport  Port=20
  FbCtl_KdVehSpdLwr_C : Inport  Port=21
  FbCtl_KdVehSpdUpr_C : Inport  Port=22
  FbCtl_KdV1_C : Inport  Port=23
  FbCtl_KdV2_C : Inport  Port=24
  FbCtl_CarWidth : Inport  Port=25
  Abs : Abs
  Add : Sum
  Add{1..2,4..5} (4 alike) : Sum  Inputs=+-
  Add3 : Sum
  Average Filter (AvrgFlt) : Subsystem
      mask Display:
      | port_label('input', 1, 'In');
      | port_label('input', 2, 'PtsNum');
      | port_label('output', 1, 'Out');
      | color('blue');
      | text(0.98,0.9,'VCDC Block','horizontalAlignment','right');
      | color('black');
      | text(0.5,0.55,'Average Filter','horizontalAlignment','center');
      | text(0.5,0.4,'(AvrgFlt)','horizontalAlignment','center');
  Bus Selector : BusSelector  OutputSignals=L0_C0
  Bus Selector1 : BusSelector  OutputSignals=R0_C0
  Constant3 : Constant  OutDataTypeStr=single
  Constant4 : Constant  Value=0.004  OutDataTypeStr=single
  Constant7 : Constant  Value=180  OutDataTypeStr=single
  Constant8 : Constant  Value=120  OutDataTypeStr=single
  Divide : Product  Inputs=*/
  Divide{1..3,7} (4 alike) : Product  Inputs=**
  Divide4 : Product  Inputs=**/
  Divide8 : Product  Inputs=**/
  Gain : Gain  Gain=-1  OutDataTypeStr=single
  Gain1 : Gain  Gain=-1
  Gain3 : Gain  Gain=-1  OutDataTypeStr=single
  Product1 : Product  OutDataTypeStr=single  RndMeth=Zero
  Product2 : Product  OutDataTypeStr=single  RndMeth=Zero
  Product4 : Product  OutDataTypeStr=single  RndMeth=Zero
  PtsNum : Constant  Value=10  OutDataTypeStr=single
  Saturable Gain Lut (SatGainLut) : MATLAB Function  TreatAsAtomicUnit=on
  Saturable Gain Lut (SatGainLut)1 : MATLAB Function  TreatAsAtomicUnit=on
  Saturation : Saturate  UpperLimit=40  LowerLimit=5
      settings: AttributesFormatString="Min = %<LowerLimit>  Max = %<UpperLimit>"
  Saturation Dynamic : simulink/Discontinuities/Saturation Dynamic  OutMin=[]  OutMax=[]  OutDataTypeStr=Inherit: Same as second input  OutDataType=fixdt(1, 16)  OutScaling=2^-10  DoSatur=off
  Saturation Dynamic2 : simulink/Discontinuities/Saturation Dynamic  OutMin=[]  OutMax=[]  OutDataTypeStr=Inherit: Same as second input  OutDataType=fixdt(1, 16)  OutScaling=2^-10  DoSatur=off
  Saturation1 : Saturate  UpperLimit=0.004  LowerLimit=0.00001
      settings: AttributesFormatString="Min = %<LowerLimit>  Max = %<UpperLimit>"
  Saturation2 : Saturate  UpperLimit=360  LowerLimit=-360  OutDataTypeStr=single
      settings: AttributesFormatString="Min = %<LowerLimit>  Max = %<UpperLimit>"
  Subsystem : Subsystem
  Subtract1 : Sum  Inputs=-+
  Subtract2 : Sum  Inputs=+-
  Switch2 : Switch
  Time : Subsystem
      mask Display:
      | port_label('output', 1, 'TTime');
      | color('blue');
      | text(0.98,0.9,'VCDC Block','horizontalAlignment','right');
      | color('black');
      | text(0.5,0.55,'Tick Time','horizontalAlignment','center');
      | text(0.5,0.4,'(TTime)','horizontalAlignment','center');
  Unit Delay : UnitDelay  SampleTime=-1
  kph to mps : Gain  Gain=1/3.6  OutDataTypeStr=single
  FbCtl_phiFbPropCtlSWA : Outport
  FbCtl_phiFbIntegCtlSWA : Outport  Port=2
  FbCtl_phiFbDiffCtlSWA : Outport  Port=3
  wires:
  Gain1/1 -> Divide7/2
  FbCtl_CarWidth/1 -> Subsystem/2(CarWidth)
  FbCtl_LaneWidth/1 -> Subsystem/1(LaneWidth)
  Saturable Gain Lut (SatGainLut)1/1(Gain) -> [FbCtl_Kd]  "Gain"
  [Vx] -> Saturable Gain Lut (SatGainLut)1/1(Input)
  FbCtl_KdV2_C/1 -> Saturable Gain Lut (SatGainLut)1/5(GainLimUpr)
  FbCtl_KdVehSpdUpr_C/1 -> Saturable Gain Lut (SatGainLut)1/3(InputLimUpr)
  FbCtl_KdVehSpdLwr_C/1 -> Saturable Gain Lut (SatGainLut)1/2(InputLimLwr)
  FbCtl_KdV1_C/1 -> Saturable Gain Lut (SatGainLut)1/4(GainLimLwr)
  FbCtl_Kp_C/1 -> Product2/2
  Product2/1 -> Saturation2/1
  FbCtl_KpKlat_C/1 -> Product1/1
  Bus Selector1/1 -> Subsystem/4(R0C0)  "<R0_C0>"
  Bus Selector/1 -> Subsystem/3(L0C0)  "<L0_C0>"
  FbCtl_bsR0Info/1 -> Bus Selector1/1
  FbCtl_bsL0Info/1 -> Bus Selector/1
  PtsNum/1 -> Average Filter (AvrgFlt)/2(PtsNum)
  Product1/1 -> Subtract1/2  "FbCtl_phiDvt"
  Average Filter (AvrgFlt)/1(Out) -> [FbCtl_phiHdAg], Subtract2/1  "FbCtl_phiHdAg"
  Saturable Gain Lut (SatGainLut)/1(Gain) -> Product4/2  "Gain"
  Saturation2/1 -> FbCtl_phiFbPropCtlSWA/1
  Saturation/1 -> Divide/2
  Divide1/1 -> Saturation/1
  FbCtl_PrvwT_C/1 -> Divide1/1
  FbCtl_PrvwDvt/1 -> Divide/1
  Divide/1 -> Product1/2
  FbCtl_PrvwHdAg/1 -> Average Filter (AvrgFlt)/1(In)
  Product4/1 -> Divide2/1, Product2/1
  kph to mps/1 -> Divide1/2, [Vx]
  FbCtl_KpVehSpdLwr_C/1 -> Saturable Gain Lut (SatGainLut)/2(InputLimLwr)
  FbCtl_KpVehSpdUpr_C/1 -> Saturable Gain Lut (SatGainLut)/3(InputLimUpr)
  FbCtl_KpV1_C1/1 -> Saturable Gain Lut (SatGainLut)/4(GainLimLwr)
  FbCtl_KpV2_C1/1 -> Saturable Gain Lut (SatGainLut)/5(GainLimUpr)
  FbCtl_Ki_C/1 -> Divide2/2
  Divide2/1 -> Switch2/3, Add/2
  Subtract1/1 -> Product4/1  "FbCtl_phiKpAg"
  Add3/1 -> Saturation Dynamic/1, Gain/1
  FbCtl_KiMaxSWA_C/1 -> Add5/1
  FbCtl_VehSpd/1 -> kph to mps/1, Saturable Gain Lut (SatGainLut)/1(Input)
  Unit Delay/1 -> Add/1
  Gain/1 -> Saturation Dynamic/3
  Saturation Dynamic/1 -> FbCtl_phiFbIntegCtlSWA/1, Unit Delay/1
  Divide7/1 -> Saturation Dynamic2/2
  Gain3/1 -> Saturation Dynamic2/3
  Divide8/1 -> Gain3/1, Saturation Dynamic2/1
  FbCtl_KdMaxSWA/1 -> Divide8/2
  Constant7/1 -> Add4/1
  Add4/1 -> Divide8/1
  Constant8/1 -> Divide8/3
  [Vx] -> Add4/2
  Subsystem/1(D) -> Divide7/1  "D"
  [FbCtl_Kd] -> Subsystem/5(FbCtl_Kd)
  Saturation Dynamic2/1 -> FbCtl_phiFbDiffCtlSWA/1
  Time/1(Out1) -> Add2/1
  [PT1] -> Add2/2
  Add2/1 -> Switch2/2
  Switch2/1 -> Saturation Dynamic/2
  Add/1 -> Switch2/1
  FbCtl_PrvwCrvt/1 -> Abs/1
  Abs/1 -> Saturation1/1
  Constant3/1 -> Add3/2, Add5/2
  Saturation1/1 -> Divide4/1
  Divide4/1 -> Add3/1
  Constant4/1 -> Divide4/3
  Add5/1 -> Divide4/2
  FbCtl_KdBalance/1 -> Subsystem/6(FbCtl_KdBalance)
  [FbCtl_phiHdAg] -> Add1/1
  Add1/1 -> Gain1/1
  Divide3/1 -> [PrvwCrvt_Comp], Add1/2
  PrvwZMean/1 -> Divide3/1
  PrvwCrvtMean/1 -> Divide3/2
  [PrvwCrvt_Comp] -> Subtract2/2
  Subtract2/1 -> Subtract1/1

== system LKAS_AutoSave_DF_20220125_0841/LKAS/LL/LLOn/LKA/Lane Following (LF)/Trajectory Following Control (TFC)/Feedforward Control (FfCtl) ==
  FfCtl_FfCtlRatio_C : Inport
  FfCtl_vVehSpd : Inport  Port=2
  FfCtl_crPrvwCrvt : Inport  Port=3
  FfCtl_lWhlBase_SY : Inport  Port=4
  FfCtl_rTraRatio_C : Inport  Port=5
  Add : Sum  OutDataTypeStr=single
  Constant : Constant  Value=0.09  OutDataTypeStr=single
  Constant1 : Constant  OutDataTypeStr=single
  Divide : Product  Inputs=*/  OutDataTypeStr=single
  Divide1 : Product  Inputs=*/  OutDataTypeStr=single
  Divide2 : Product  Inputs=*/
  Gain2 : Gain  Gain=-1  OutDataTypeStr=single
  Math Function : Math  Operator=magnitude^2  OutDataTypeStr=single  SaturateOnIntegerOverflow=on
  Product : Product  OutDataTypeStr=single
  Product1 : Product  OutDataTypeStr=single
  Product2 : Product  OutDataTypeStr=single
  Product3 : Product  Inputs=3  OutDataTypeStr=single
  Saturation1 : Saturate  UpperLimit=0.01  LowerLimit=0
      settings: AttributesFormatString="Min = %<LowerLimit>  Max = %<UpperLimit>"
  Saturation3 : Saturate  UpperLimit=150  LowerLimit=60
      settings: AttributesFormatString="Min = %<LowerLimit>  Max = %<UpperLimit>"
  kph to mps : Gain  Gain=1/3.6  OutDataTypeStr=single
  rad to deg : Gain  Gain=180/pi  OutDataTypeStr=single
  FfCtl_phiFfSWA : Outport
  wires:
  Gain2/1 -> FfCtl_phiFfSWA/1
  kph to mps/1 -> Divide/1, Math Function/1, Product/1
  rad to deg/1 -> Product1/1
  Product1/1 -> Product3/2
  Divide1/1 -> Product1/2
  Divide/1 -> Divide1/2
  FfCtl_lWhlBase_SY/1 -> Divide/2
  Add/1 -> Divide1/1
  Constant1/1 -> Add/2
  Product2/1 -> Add/1
  Math Function/1 -> Product2/1
  Product/1 -> rad to deg/1
  FfCtl_crPrvwCrvt/1 -> Product/2
  FfCtl_vVehSpd/1 -> Saturation3/1, kph to mps/1
  Product3/1 -> Gain2/1
  FfCtl_rTraRatio_C/1 -> Product3/3
  FfCtl_FfCtlRatio_C/1 -> Product3/1
  Divide2/1 -> Saturation1/1
  Saturation1/1 -> Product2/2  "FfCtl_facmUSG_C"
  Constant/1 -> Divide2/1
  Saturation3/1 -> Divide2/2  "Vx"

== system LKAS_AutoSave_DF_20220125_0841/LKAS/LL/LLOn/LKA/Plan To LaneFollowing (PTLF)/InsideJudge1/If Action Subsystem ==
  T1 : Inport
  Plan : Inport  Port=2
  HdAgLft : Inport  Port=3
  Time : Inport  Port=4
  Action Port : ActionPort  InitializeStates=reset
      settings: AttributesFormatString=states = %<InitializeStates>
  Add : Sum
  Cast To Single : DataTypeConversion  OutDataTypeStr=uint8
  Compare To Constant : simulink/Logic and Bit Operations/Compare To Constant  relop=>=  const=0  OutDataTypeStr=boolean
  Detect Decrease : simulink/Logic and Bit Operations/Detect Decrease  vinit=0.0  OutDataTypeStr=boolean
  If Action Subsystem : Subsystem  TreatAsAtomicUnit=on
  If Action Subsystem2 : Subsystem  TreatAsAtomicUnit=on
  Logical Operator : Logic  AllPortsSameDT=off  OutDataTypeStr=boolean
  Memory : Memory  InheritSampleTime=on
  Relational Operator : RelationalOperator  OutDataTypeStr=boolean  RndMeth=Simplest
  Saturation : Saturate  UpperLimit=5  LowerLimit=0
      settings: AttributesFormatString="Min = %<LowerLimit>  Max = %<UpperLimit>"
  Switch : Switch  Criteria=u2 > Threshold
  Switch1 : Switch  Criteria=u2 > Threshold
  T1_1 : Outport
      settings: AttributesFormatString=%<OutputWhenDisabled> = %<InitialOutput>
  Plan_1 : Outport  Port=2
      settings: AttributesFormatString=%<OutputWhenDisabled> = %<InitialOutput>
  wires:
  HdAgLft/1 -> Compare To Constant/1
  Compare To Constant/1 -> Detect Decrease/1
  Time/1 -> If Action Subsystem/1(T1), Relational Operator/2
  Plan/1 -> If Action Subsystem2/2(Plan), If Action Subsystem/2(Plan)
  T1/1 -> If Action Subsystem2/1(T1), Relational Operator/1
  Detect Decrease/1 -> Logical Operator/1
  Relational Operator/1 -> Logical Operator/2
  Add/1 -> Saturation/1
  Memory/1 -> Add/2
  Logical Operator/1 -> Cast To Single/1
  Cast To Single/1 -> Add/1
  Saturation/1 -> Switch1/2, Switch/2, If Action Subsystem/Enable, Memory/1
  If Action Subsystem/1(T1_1) -> Switch/1
  If Action Subsystem/2(Plan_1) -> Switch1/1
  If Action Subsystem2/1(T1_1) -> Switch/3
  If Action Subsystem2/2(Plan_1) -> Switch1/3
  Switch/1 -> T1_1/1
  Switch1/1 -> Plan_1/1

== system LKAS_AutoSave_DF_20220125_0841/LKAS/LL/LLOn/LKA/Plan To LaneFollowing (PTLF)/InsideJudge1/If Action Subsystem1 ==
  T1 : Inport
  Plan : Inport  Port=2
  HdAgRgt : Inport  Port=3
  Time : Inport  Port=4
  Action Port : ActionPort  InitializeStates=reset
      settings: AttributesFormatString=states = %<InitializeStates>
  Add : Sum
  Cast To Single : DataTypeConversion  OutDataTypeStr=uint8
  Compare To Constant : simulink/Logic and Bit Operations/Compare To Constant  relop=<=  const=0  OutDataTypeStr=boolean
  Detect Decrease : simulink/Logic and Bit Operations/Detect Decrease  vinit=0.0  OutDataTypeStr=boolean
  If Action Subsystem : Subsystem  TreatAsAtomicUnit=on
  If Action Subsystem2 : Subsystem  TreatAsAtomicUnit=on
  Logical Operator : Logic  AllPortsSameDT=off  OutDataTypeStr=boolean
  Memory : Memory  InheritSampleTime=on
  Relational Operator : RelationalOperator  OutDataTypeStr=boolean  RndMeth=Simplest
  Saturation : Saturate  UpperLimit=5  LowerLimit=0
      settings: AttributesFormatString="Min = %<LowerLimit>  Max = %<UpperLimit>"
  Switch : Switch  Criteria=u2 > Threshold
  Switch1 : Switch  Criteria=u2 > Threshold
  T1_1 : Outport
      settings: AttributesFormatString=%<OutputWhenDisabled> = %<InitialOutput>
  Plan_1 : Outport  Port=2
      settings: AttributesFormatString=%<OutputWhenDisabled> = %<InitialOutput>
  wires:
  Relational Operator/1 -> Logical Operator/2
  Detect Decrease/1 -> Logical Operator/1
  Compare To Constant/1 -> Detect Decrease/1
  HdAgRgt/1 -> Compare To Constant/1
  Time/1 -> Relational Operator/2, If Action Subsystem/1(T1)
  Add/1 -> Saturation/1
  T1/1 -> If Action Subsystem2/1(T1), Relational Operator/1
  Memory/1 -> Add/2
  Logical Operator/1 -> Cast To Single/1
  Cast To Single/1 -> Add/1
  Saturation/1 -> Memory/1, Switch1/2, Switch/2, If Action Subsystem/Enable
  If Action Subsystem2/1(T1_1) -> Switch/3
  If Action Subsystem/2(Plan_1) -> Switch1/1
  Switch/1 -> T1_1/1
  Switch1/1 -> Plan_1/1
  If Action Subsystem2/2(Plan_1) -> Switch1/3
  If Action Subsystem/1(T1_1) -> Switch/1
  Plan/1 -> If Action Subsystem/2(Plan), If Action Subsystem2/2(Plan)

== system LKAS_AutoSave_DF_20220125_0841/LKAS/LL/LLOn/LKA/Plan To LaneFollowing (PTLF)/InsideJudge1/If Action Subsystem2 ==
  T1 : Inport
  Plan : Inport  Port=2
  Action Port : ActionPort  InitializeStates=reset
      settings: AttributesFormatString=states = %<InitializeStates>
  T1_1 : Outport
      settings: AttributesFormatString=%<OutputWhenDisabled> = %<InitialOutput>
  Plan_1 : Outport  Port=2
      settings: AttributesFormatString=%<OutputWhenDisabled> = %<InitialOutput>
  wires:
  T1/1 -> T1_1/1
  Plan/1 -> Plan_1/1

== system LKAS_AutoSave_DF_20220125_0841/LKAS/LL/LLOn/LKA Input Processing (LKAInP)/Previewed Curvature Calculation (PrCrvt)/Lane Information Selection (LaneInfoSel)/If Action Subsystem1 ==
  In1 : Inport
  Action Port : ActionPort  InitializeStates=reset
      settings: AttributesFormatString=states = %<InitializeStates>
  Out1 : Outport
      settings: AttributesFormatString=%<OutputWhenDisabled> = %<InitialOutput>
  wires:
  In1/1 -> Out1/1

== system LKAS_AutoSave_DF_20220125_0841/LKAS/LL/LLOn/LKA Input Processing (LKAInP)/Previewed Curvature Calculation (PrCrvt)/Lane Information Selection (LaneInfoSel)/If Action Subsystem2 ==
  In1 : Inport
  Action Port : ActionPort  InitializeStates=reset
      settings: AttributesFormatString=states = %<InitializeStates>
  Out1 : Outport
      settings: AttributesFormatString=%<OutputWhenDisabled> = %<InitialOutput>
  wires:
  In1/1 -> Out1/1

== system LKAS_AutoSave_DF_20220125_0841/LKAS/LL/LLOn/LKA Input Processing (LKAInP)/Previewed Curvature Calculation (PrCrvt)/Lane Information Selection (LaneInfoSel)/If Action Subsystem3 ==
  In1 : Inport
  In2 : Inport  Port=2
  Action Port : ActionPort  InitializeStates=reset
      settings: AttributesFormatString=states = %<InitializeStates>
  Add : Sum
  Gain : Gain  Gain=0.5
  Out1 : Outport
      settings: AttributesFormatString=%<OutputWhenDisabled> = %<InitialOutput>
  wires:
  Gain/1 -> Out1/1
  In1/1 -> Add/1
  In2/1 -> Add/2
  Add/1 -> Gain/1

== system LKAS_AutoSave_DF_20220125_0841/LKAS/LL/LLOn/LKA Input Processing (LKAInP)/Steering Wheel Position Calculation (SWAPosCal)/Subsystem/LowPass ==
  T : Inport
  u : Inport  Port=2
  dT : Inport  Port=3
  Add : Sum  Inputs=+-
  Add1 : Sum
  Add2 : Sum  OutDataTypeStr=single
  Divide : Product  Inputs=*/
  Divide1 : Product  Inputs=**
  Memory3 : Memory  InheritSampleTime=on
  SWACmdSyn_tiSmplT_C4 : Constant  OutDataTypeStr=single
  Saturation : Saturate  UpperLimit=50  LowerLimit=0
      settings: AttributesFormatString="Min = %<LowerLimit>  Max = %<UpperLimit>"
  Switch : Switch  Criteria=u2 > Threshold  Threshold=1
  Unit Delay : UnitDelay  SampleTime=-1
  y : Outport
  wires:
  Switch/1 -> Unit Delay/1, y/1
  Memory3/1 -> Add2/2
  Saturation/1 -> Memory3/1, Switch/2
  Add2/1 -> Saturation/1
  SWACmdSyn_tiSmplT_C4/1 -> Add2/1
  Add1/1 -> Switch/1
  Unit Delay/1 -> Add1/2, Add/2
  Divide1/1 -> Add1/1
  Add/1 -> Divide1/2
  Divide/1 -> Divide1/1
  u/1 -> Add/1, Switch/3
  dT/1 -> Divide/1
  T/1 -> Divide/2

== system LKAS_AutoSave_DF_20220125_0841/LKAS/LL/LLOn/LKA Input Processing (LKAInP)/Steering Wheel Position Calculation (SWAPosCal)/Subsystem1/Subsystem ==
  In : Inport
  In1 : Inport  Port=2
  Enable : EnablePort  StatesWhenEnabling=reset
      settings: AttributesFormatString=states = %<StatesWhenEnabling>
  Add1 : Sum  OutDataTypeStr=uint16
  Cast To Single : DataTypeConversion  OutDataTypeStr=uint16
  Cast To Single1 : DataTypeConversion  OutDataTypeStr=uint16
  Memory : Memory  InheritSampleTime=on
  Relational Operator : RelationalOperator  OutDataTypeStr=boolean  RndMeth=Nearest
  Saturation : Saturate  UpperLimit=3000  LowerLimit=0  OutDataTypeStr=uint16
      settings: AttributesFormatString="Min = %<LowerLimit>  Max = %<UpperLimit>"
  Out : Outport  OutputWhenDisabled=reset  InitialOutput=0
      settings: AttributesFormatString=%<OutputWhenDisabled> = %<InitialOutput>
  wires:
  Cast To Single1/1 -> Relational Operator/2
  In/1 -> Cast To Single/1
  Relational Operator/1 -> Out/1
  In1/1 -> Cast To Single1/1
  Cast To Single/1 -> Add1/1
  Memory/1 -> Add1/2
  Saturation/1 -> Relational Operator/1, Memory/1
  Add1/1 -> Saturation/1

== system LKAS_AutoSave_DF_20220125_0841/LKAS/LL/LLOn/LL State Determination (LLStateDet)/LL State Machine Conditions (LLSMCon)/Activation Condition (ActvC)/Activation Condition Synthesis (ActvCSyn) ==
  ActvCSyn_stDACMode : Inport
  ActvCSyn_stEPSCtlEC : Inport  Port=2
  ActvCSyn_stDvtThresActvFlgLDW : Inport  Port=3
  ActvCSyn_stDvtThresActvFlgLKA : Inport  Port=4
  ActvCSyn_stLaneQlECFlg : Inport  Port=5
  Default Flag (DflFlg) : Subsystem  TreatAsAtomicUnit=on
  Default Flag (DflFlg)1 : Subsystem  TreatAsAtomicUnit=on
  If : If  NumInputs=3  IfExpression=(u1 ==1|u1==2)& u2 == 1 & u3 == 1  ElseIfExpressions=(u1 ==1|u1==2)& u2 == 2 & u3 == 1
  If1 : If  NumInputs=4  IfExpression=u1 == 2 & u2 == 1 & u3 == 1 & u4 == 1  ElseIfExpressions=u1 == 2 & u2 == 2 & u3 == 1 & u4 == 1
  LDW Left Active Flag (LDWLftActvFlg) : Subsystem  TreatAsAtomicUnit=on
  LDW Right Active Flag (LDWRgtActvFlg) : Subsystem  TreatAsAtomicUnit=on
  LKA Left Active Flag (LKALftActvFlg)1 : Subsystem  TreatAsAtomicUnit=on
  LKA Right Active Flag (LKARgtActvFlg)1 : Subsystem  TreatAsAtomicUnit=on
  Merge : Merge  Inputs=3
  Merge2 : Merge  Inputs=3
  ActvCSyn_stLDWActvCSyn : Outport
  ActvCSyn_stLKAActvCSyn : Outport  Port=2
  wires:
  LDW Left Active Flag (LDWLftActvFlg)/1(Out) -> Merge/1
  If/1 -> LDW Left Active Flag (LDWLftActvFlg)/Action
  If/3 -> Default Flag (DflFlg)/Action
  If/2 -> LDW Right Active Flag (LDWRgtActvFlg)/Action
  ActvCSyn_stDACMode/1 -> If1/1, If/1
  LDW Right Active Flag (LDWRgtActvFlg)/1(Out) -> Merge/2
  Merge/1 -> ActvCSyn_stLDWActvCSyn/1
  If1/3 -> Default Flag (DflFlg)1/Action
  Default Flag (DflFlg)/1(Out) -> Merge/3
  Merge2/1 -> ActvCSyn_stLKAActvCSyn/1
  LKA Left Active Flag (LKALftActvFlg)1/1(Out) -> Merge2/1
  If1/1 -> LKA Left Active Flag (LKALftActvFlg)1/Action
  LKA Right Active Flag (LKARgtActvFlg)1/1(Out) -> Merge2/2
  If1/2 -> LKA Right Active Flag (LKARgtActvFlg)1/Action
  Default Flag (DflFlg)1/1(Out) -> Merge2/3
  ActvCSyn_stEPSCtlEC/1 -> If1/3
  ActvCSyn_stDvtThresActvFlgLKA/1 -> If1/2
  ActvCSyn_stLaneQlECFlg/1 -> If/3, If1/4
  ActvCSyn_stDvtThresActvFlgLDW/1 -> If/2

== system LKAS_AutoSave_DF_20220125_0841/LKAS/LL/LLOn/LL State Determination (LLStateDet)/LL State Machine Conditions (LLSMCon)/Activation Condition (ActvC)/Deviation Threshold Condition (DvtThresCon) ==
  DvtThresCon_lLaneWidth : Inport
  DvtThresCon_ILftDvt : Inport  Port=2
  DvtThresCon_IRgtDvt : Inport  Port=3
  DvtThresCon_bsDvtThresClb : Inport  Port=4
  DvtThresCon_InInfoSyn : Inport  Port=5
  Active Lane Calculation (ActLanCalc) : Subsystem
  Bus Selector1 : BusSelector  OutputSignals=bsLaneInfo.bsL0Info.L0_C1,bsVehMovInfo.ESC_VehSpd,bsLaneInfo.bsR0Info.R0_C1
  Deviation Threshold Judgement LDW (DvtThresJdg) : Subsystem
  Deviation Threshold Judgement LKA (DvtThresJdg) : Subsystem
  Divide : Product  Inputs=**  OutDataTypeStr=single
  Divide1 : Product  Inputs=**  OutDataTypeStr=single
  Gain : Gain  Gain=1/3.6  OutDataTypeStr=single
  Saturation1 : Saturate  UpperLimit=2  LowerLimit=-2
      settings: AttributesFormatString="Min = %<LowerLimit>  Max = %<UpperLimit>"
  Saturation5 : Saturate  UpperLimit=2  LowerLimit=-2
      settings: AttributesFormatString="Min = %<LowerLimit>  Max = %<UpperLimit>"
  DvtThresCon_stDvtThresActvFlgLDW : Outport
  DvtThresCon_stDvtThresActvFlgLKA : Outport  Port=2
  wires:
  DvtThresCon_InInfoSyn/1 -> Bus Selector1/1
  Divide1/1 -> Deviation Threshold Judgement LDW (DvtThresJdg)/4(DvtThresJdg_vRgtDvtSpd), Deviation Threshold Judgement LKA (DvtThresJdg)/4(DvtThresJdg_vRgtDvtSpd)
  Divide/1 -> Deviation Threshold Judgement LKA (DvtThresJdg)/3(DvtThresJdg_vLftDvtSpd), Deviation Threshold Judgement LDW (DvtThresJdg)/3(DvtThresJdg_vLftDvtSpd)
  Gain/1 -> Divide1/1, Divide/2
  Bus Selector1/2 -> Gain/1  "<ESC_VehSpd>"
  Bus Selector1/1 -> Divide/1  "<L0_C1>"
  Bus Selector1/3 -> Divide1/2  "<R0_C1>"
  DvtThresCon_lLaneWidth/1 -> Active Lane Calculation (ActLanCalc)/1(ActLanCalc_lLaneWidth)
  DvtThresCon_ILftDvt/1 -> Saturation5/1  "DvtCalc_lLftDvt"
  DvtThresCon_IRgtDvt/1 -> Saturation1/1  "DvtCalc_lRgtDvt"
  Deviation Threshold Judgement LKA (DvtThresJdg)/1(DvtThresJdg_stDvtThresActvFlg) -> DvtThresCon_stDvtThresActvFlgLKA/1  "DvtThresActvFlg"
  Active Lane Calculation (ActLanCalc)/1(ActLanCalc_ActvCClbOut) -> Deviation Threshold Judgement LKA (DvtThresJdg)/5(DvtThresJdg_bsDvtThresClb), Deviation Threshold Judgement LDW (DvtThresJdg)/5(DvtThresJdg_bsDvtThresClb)
  Saturation5/1 -> Deviation Threshold Judgement LDW (DvtThresJdg)/1(DvtThresJdg_lLftDvt), Deviation Threshold Judgement LKA (DvtThresJdg)/1(DvtThresJdg_lLftDvt)
  Saturation1/1 -> Deviation Threshold Judgement LDW (DvtThresJdg)/2(DvtThresJdg_lRgtDvt), Deviation Threshold Judgement LKA (DvtThresJdg)/2(DvtThresJdg_lRgtDvt)
  Deviation Threshold Judgement LDW (DvtThresJdg)/1(DvtThresJdg_stDvtThresActvFlg) -> DvtThresCon_stDvtThresActvFlgLDW/1  "DvtThresActvFlg"
  DvtThresCon_bsDvtThresClb/1 -> Active Lane Calculation (ActLanCalc)/2(ActLanCalc_Clb)
